simulink model "SCIM02"  (R2016a)
settings: Solver=FixedStepAuto  StartTime=0.0  StopTime=10  FixedStep=0.0001  RelTol=1e-3
values from neighbouring files (symbols this model uses):
  Lm = 0.1271    [motor4_workspace.mat]    (also in motor_wrapper.m = obj.Lm; scim_verifier.m = obj.motor.getLm(); setMotorParams.m; stationary_class.m = obj.Lm)
  Lr = 0.2744    [motor4_workspace.mat]    (also in motor_wrapper.m = obj.Lr; scim_verifier.m = obj.motor.getLr(); setMotorParams.m; stationary_class.m = obj.Lr)
  Ls = 0.2744    [motor4_workspace.mat]    (also in motor_wrapper.m = obj.Ls; scim_verifier.m = obj.motor.getLs(); setMotorParams.m; stationary.m = Ls/10)
  Rr = 1.009    [motor4_workspace.mat]    (also in motor_wrapper.m = obj.Rr; setMotorParams.m; stationary_class.m = obj.Rr; stationary_from_eq.m = obj.Rr)
  sig = (tox-fromx)/6    [gaussSpace.m]    (also in motor4_workspace.mat = 0.785452782217; setMotorParams.m = 0.785452782217; stationary_class.m = 1-Lm*Lm/Ls/Lr; torqueFinder.m = 0.785452782217)
settings Model: Creator=ebenera  LastModifiedBy=ebenera

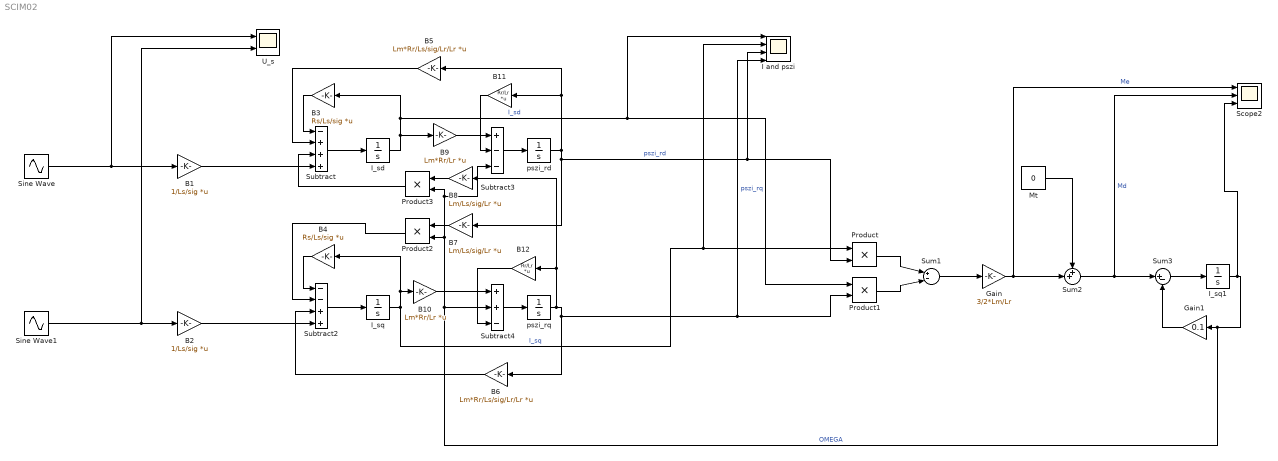
== system SCIM02 ==
  B1 : Gain  Gain=1/Ls/sig  Multiplication=Matrix(K*u)
  B10 : Gain  Gain=Lm*Rr/Lr  Multiplication=Matrix(K*u)
  B11 : Gain  Gain=Rr/Lr  Multiplication=Matrix(K*u)
  B12 : Gain  Gain=Rr/Lr  Multiplication=Matrix(K*u)
  B2 : Gain  Gain=1/Ls/sig  Multiplication=Matrix(K*u)
  B3 : Gain  Gain=Rs/Ls/sig  Multiplication=Matrix(K*u)
  B4 : Gain  Gain=Rs/Ls/sig  Multiplication=Matrix(K*u)
  B5 : Gain  Gain=Lm*Rr/Ls/sig/Lr/Lr  Multiplication=Matrix(K*u)
  B6 : Gain  Gain=Lm*Rr/Ls/sig/Lr/Lr  Multiplication=Matrix(K*u)
  B7 : Gain  Gain=Lm/Ls/sig/Lr  Multiplication=Matrix(K*u)
  B8 : Gain  Gain=Lm/Ls/sig/Lr  Multiplication=Matrix(K*u)
  B9 : Gain  Gain=Lm*Rr/Lr  Multiplication=Matrix(K*u)
  Gain : Gain  Gain=3/2*Lm/Lr
  Gain1 : Gain  Gain=0.1
  I and pszi : Scope  NumInputPorts=4
  I_sd : Integrator
  I_sq : Integrator
  I_sq1 : Integrator
  Mt : Constant  Value=0
  Product{,1..3} (4 alike) : Product
  Scope2 : Scope  NumInputPorts=3
  Sine Wave : Sin  Amplitude=8  Frequency=314  SampleTime=0
  Sine Wave1 : Sin  Amplitude=8  Frequency=314  Phase=1.5  SampleTime=0
  Subtract : Sum  Inputs=-+++
  Subtract2 : Sum  Inputs=--++
  Subtract3 : Sum  Inputs=+--
  Subtract4 : Sum  Inputs=++-
  Sum1 : Sum  Inputs=|+-|
  Sum2 : Sum  Inputs=++|
  Sum3 : Sum  Inputs=|+-
  U_s : Scope  NumInputPorts=2
  pszi_rd : Integrator
  "pszi_rq " : Integrator
  wires:
  Sine Wave1/1 -> U_s/2, B2/1
  I_sd/1 -> B9/1, I and pszi/1, Product1/1, B3/1  "I_sd"
  I_sq/1 -> B10/1, B4/1, I and pszi/2, Product/1  "I_sq"
  pszi_rd/1 -> I and pszi/3, Product/2, B7/1, B11/1, B5/1  "pszi_rd"
  "pszi_rq "/1 -> I and pszi/4, Product1/2, B6/1, B12/1, B8/1  "pszi_rq"
  Product/1 -> Sum1/1
  Product1/1 -> Sum1/2
  Sum1/1 -> Gain/1
  Gain/1 -> Scope2/1, Sum2/2  "Me"
  Mt/1 -> Sum2/1
  Sum2/1 -> Scope2/2, Sum3/1  "Md"
  Gain1/1 -> Sum3/2
  Sum3/1 -> I_sq1/1
  I_sq1/1 -> Scope2/3, Subtract4/2, Subtract3/3, Product3/2, Product2/2, Gain1/1  "OMEGA"
  Subtract/1 -> I_sd/1
  Sine Wave/1 -> U_s/1, B1/1
  B2/1 -> Subtract2/4
  B1/1 -> Subtract/4
  Subtract2/1 -> I_sq/1
  B3/1 -> Subtract/1
  B4/1 -> Subtract2/1
  B5/1 -> Subtract/2
  B6/1 -> Subtract2/3
  B7/1 -> Product2/1
  Product2/1 -> Subtract2/2
  B8/1 -> Product3/1
  Product3/1 -> Subtract/3
  Subtract3/1 -> pszi_rd/1
  Subtract4/1 -> "pszi_rq "/1
  B9/1 -> Subtract3/1
  B10/1 -> Subtract4/1
  B11/1 -> Subtract3/2
  B12/1 -> Subtract4/3
